simulink model "Estimare_perturbatie"  (R2020b)
settings: Solver=VariableStepAuto  StartTime=0.0  StopTime=4.5  RelTol=1e-3
values from neighbouring files (symbols this model uses):
  Ad = eye(size(A))+Ts*A    [Script_pendul.m]
  Ae = [Ad E;zeros(1,nstates),ones(1,nperturbatii)]    [Script_pendul.m]
  Bd = Ts*B    [Script_pendul.m]
  Be = [Bd;zeros(1,nperturbatii)]    [Script_pendul.m]
  Cd = C    [Script_pendul.m]
  Ce = [Cd,zeros(noutputs,nperturbatii)]    [Script_pendul.m]
  E = [0.5 0 0.1 0]'    [Script_pendul.m]
  Le = Le'    [Script_pendul.m]
  Ts = 0.001    [Script_pendul.m]
libraries: eeStairGenerator x1
settings Model: Creator=tudor  LastModifiedBy=tudor

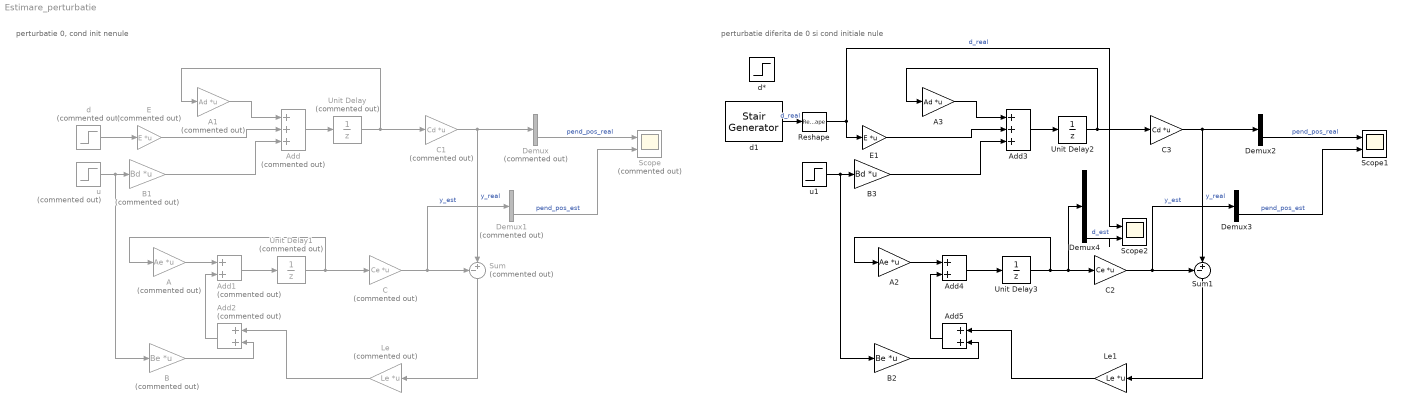
== system Estimare_perturbatie ==
  note: perturbatie 0, cond init nenule
  note: perturbatie diferita de 0 si cond initiale nule
  A : Gain  Commented=on  Gain=Ae  Multiplication=Matrix(K*u)
  A1 : Gain  Commented=on  Gain=Ad  Multiplication=Matrix(K*u)
  A2 : Gain  Gain=Ae  Multiplication=Matrix(K*u)
  A3 : Gain  Gain=Ad  Multiplication=Matrix(K*u)
  Add : Sum  Commented=on  Inputs=+++
  Add1 : Sum  Commented=on
  Add2 : Sum  Commented=on
  Add3 : Sum  Inputs=+++
  Add4 : Sum
  Add5 : Sum
  B : Gain  Commented=on  Gain=Be  Multiplication=Matrix(K*u)
  B1 : Gain  Commented=on  Gain=Bd  Multiplication=Matrix(K*u)
  B2 : Gain  Gain=Be  Multiplication=Matrix(K*u)
  B3 : Gain  Gain=Bd  Multiplication=Matrix(K*u)
  C : Gain  Commented=on  Gain=Ce  Multiplication=Matrix(K*u)
  C1 : Gain  Commented=on  Gain=Cd  Multiplication=Matrix(K*u)
  C2 : Gain  Gain=Ce  Multiplication=Matrix(K*u)
  C3 : Gain  Gain=Cd  Multiplication=Matrix(K*u)
  Demux : Demux  Commented=on  Outputs=2
  Demux1 : Demux  Commented=on  Outputs=2
  Demux2 : Demux  Outputs=2
  Demux3 : Demux  Outputs=2
  Demux4 : Demux  Outputs=5
  E : Gain  Commented=on  Gain=E  Multiplication=Matrix(K*u)
  E1 : Gain  Gain=E  Multiplication=Matrix(K*u)
  Le : Gain  Commented=on  Gain=Le  Multiplication=Matrix(K*u)
  Le1 : Gain  Gain=Le  Multiplication=Matrix(K*u)
  Reshape : Reshape
  Scope : Scope  Commented=on  NumInputPorts=2
  Scope1 : Scope  NumInputPorts=2
  Scope2 : Scope  NumInputPorts=2
  Sum : Sum  Commented=on  Inputs=-+|
  Sum1 : Sum  Inputs=-+|
  Unit Delay : UnitDelay  Commented=on  InitialCondition=[0 0 0.05 0]  SampleTime=Ts  HasFrameUpgradeWarning=on
  Unit Delay1 : UnitDelay  Commented=on  InitialCondition=[0 0 0.5 0 0]  SampleTime=Ts  HasFrameUpgradeWarning=on
  Unit Delay2 : UnitDelay  InitialCondition=[0 0 0 0]  SampleTime=Ts  HasFrameUpgradeWarning=on
  Unit Delay3 : UnitDelay  InitialCondition=[0 0 0.5 0 0]  SampleTime=Ts  HasFrameUpgradeWarning=on
  d : Step  Commented=on  Time=0  After=0  SampleTime=Ts
  d* : Step  Time=4  After=0.1  SampleTime=0
  d1 : eeStairGenerator/Stair Generator  LabelModeActiveChoice=Discrete  TimeInput=[0 1 3]  AmplitudeInput=[0 0.1 -0.3]  SampleTime=Ts  RepeatPattern=off  OutDataTypeStr=double
      settings: SourceProductBaseCode=PS
  u : Step  Commented=on  Time=0  After=0  SampleTime=Ts
  u1 : Step  Time=0  After=0  SampleTime=Ts
  wires:
  A1/1 -> Add/1
  E/1 -> Add/2
  Unit Delay/1 -> A1/1, C1/1
  Add/1 -> Unit Delay/1
  d/1 -> E/1
  u/1 -> B/1, B1/1
  B1/1 -> Add/3
  A/1 -> Add1/1
  Add1/1 -> Unit Delay1/1
  Unit Delay1/1 -> A/1, C/1
  C/1 -> Demux1/1, Sum/1  "y_est"
  C1/1 -> Sum/2, Demux/1  "y_real"
  Sum/1 -> Le/1
  Le/1 -> Add2/1
  B/1 -> Add2/2
  Add2/1 -> Add1/2
  Demux/2 -> Scope/1  "pend_pos_real"
  Demux1/2 -> Scope/2  "pend_pos_est"
  B2/1 -> Add5/2
  Add4/1 -> Unit Delay3/1
  Unit Delay3/1 -> A2/1, Demux4/1, C2/1
  Demux3/2 -> Scope1/2  "pend_pos_est"
  A2/1 -> Add4/1
  Unit Delay2/1 -> C3/1, A3/1
  Add3/1 -> Unit Delay2/1
  u1/1 -> B2/1, B3/1
  E1/1 -> Add3/2
  Reshape/1 -> Scope2/1, E1/1  "d_real"
  A3/1 -> Add3/1
  Sum1/1 -> Le1/1
  Demux2/2 -> Scope1/1  "pend_pos_real"
  C3/1 -> Sum1/2, Demux2/1  "y_real"
  Le1/1 -> Add5/1
  C2/1 -> Demux3/1, Sum1/1  "y_est"
  Add5/1 -> Add4/2
  B3/1 -> Add3/3
  Demux4/5 -> Scope2/2  "d_est"
  d1/1 -> Reshape/1  "d_real"
